simulink model "Engine"  (Simulink 9.3)
settings: Solver=ode23tb  StartTime=0.0  StopTime=50  FixedStep=0.001  EnableMultiTasking=on
values from neighbouring files (symbols this model uses):
  toggle_paf = toggle(2)    [RunEngine.m]
  toggle_vol = toggle(3)    [RunEngine.m]
  toggle_Waf = toggle(4)    [RunEngine.m]
  toggle_Wc = toggle(5)    [RunEngine.m]
  toggle_Wic = toggle(6)    [RunEngine.m]
  toggle_Wth = toggle(7)    [RunEngine.m]
  toggle_xth = toggle(8)    [RunEngine.m]
  toggle_ypic = toggle(9)    [RunEngine.m]
  toggle_ypim = toggle(10)    [RunEngine.m]
  toggle_yTic = toggle(11)    [RunEngine.m]
  toggle_yWaf = toggle(12)    [RunEngine.m]
undefined symbols (not defined in the file or in its folder): a0, a1, a2, dP_thrREF, KpThr, KpWg, n_r, Newton, r_c, Raphson, T_z, TC_ENGINE, TiThr, TiWg
libraries: simulink x3
(part 3 of 3)

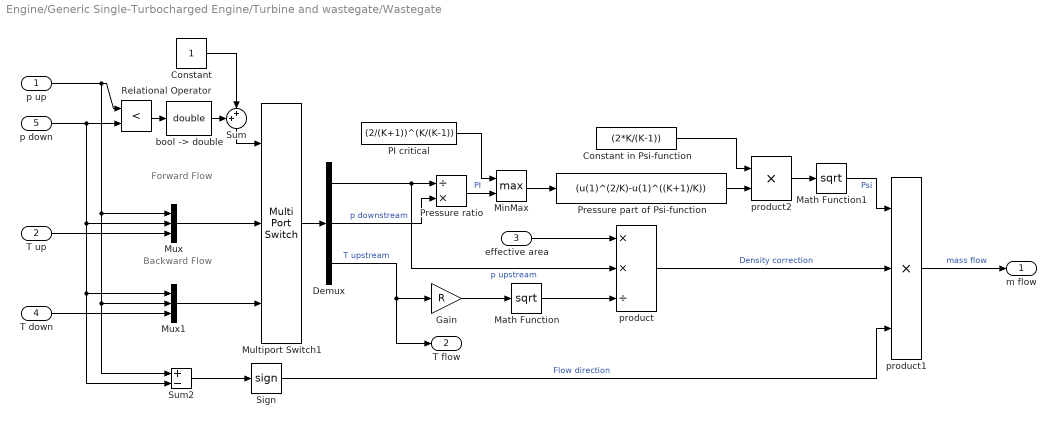
== system Engine/Generic Single-Turbocharged Engine/Turbine and wastegate/Wastegate ==
  note: Forward
      | Flow
  note: Backward
      | Flow
  p up : Inport
  T up : Inport  Port=2
  effective area : Inport  Port=3
  T down : Inport  Port=4
  p down : Inport  Port=5
  Constant : Constant
  Constant in Psi-function : Constant  Value=(2*K/(K-1))
  Demux : Demux  Outputs=3
  Gain : Gain  Gain=R  SaturateOnIntegerOverflow=on  OutDataTypeStr=Inherit: Same as input  ParamDataTypeStr=Inherit: Same as input
  Math Function : Math  Operator=sqrt  SaturateOnIntegerOverflow=on
  Math Function1 : Math  Operator=sqrt  SaturateOnIntegerOverflow=on
  MinMax : MinMax  Function=max  Inputs=2  ZeroCross=off  SaturateOnIntegerOverflow=on  InputSameDT=on
  Multiport Switch1 : MultiPortSwitch  Inputs=2  SaturateOnIntegerOverflow=on  InputSameDT=on
  Mux : Mux  Inputs=3
  Mux1 : Mux  Inputs=3
  PI critical : Constant  Value=(2/(K+1))^(K/(K-1))
  Pressure ratio : Product  Inputs=/*  SaturateOnIntegerOverflow=on  InputSameDT=on  OutDataTypeStr=Inherit: Same as first input
  Pressure part of Psi-function : Fcn  Expr=(u(1)^(2/K)-u(1)^((K+1)/K))
  Relational Operator : RelationalOperator  Operator=<  RndMeth=Nearest  InputSameDT=on
  Sign : Signum  ZeroCross=off
  Sum : Sum  Inputs=++|  SaturateOnIntegerOverflow=on  InputSameDT=on  OutDataTypeStr=Inherit: Same as first input
  Sum2 : Sum  Inputs=+-  SaturateOnIntegerOverflow=on  InputSameDT=on  OutDataTypeStr=Inherit: Same as first input
  "bool -> double" : DataTypeConversion  OutDataTypeStr=double  SaturateOnIntegerOverflow=on  RndMeth=Zero
  product : Product  Inputs=**/  SaturateOnIntegerOverflow=on  InputSameDT=on  OutDataTypeStr=Inherit: Same as first input
  product1 : Product  Inputs=3  SaturateOnIntegerOverflow=on  InputSameDT=on  OutDataTypeStr=Inherit: Same as first input
  product2 : Product  SaturateOnIntegerOverflow=on  InputSameDT=on  OutDataTypeStr=Inherit: Same as first input
  m flow : Outport
  T flow : Outport  Port=2
  wires:
  "bool -> double"/1 -> Sum/1
  Demux/3 -> T flow/1, Gain/1  "T upstream"
  Math Function1/1 -> product1/1  "Psi"
  product2/1 -> Math Function1/1
  Sign/1 -> product1/3  "Flow direction"
  product/1 -> product1/2  "Density correction"
  Pressure part of Psi-function/1 -> product2/2
  Constant in Psi-function/1 -> product2/1
  Math Function/1 -> product/3
  Gain/1 -> Math Function/1
  Demux/1 -> product/2, Pressure ratio/1  "p upstream"
  effective area/1 -> product/1
  product1/1 -> m flow/1  "mass flow"
  MinMax/1 -> Pressure part of Psi-function/1
  PI critical/1 -> MinMax/1
  Pressure ratio/1 -> MinMax/2  "PI"
  Sum2/1 -> Sign/1
  Demux/2 -> Pressure ratio/2  "p downstream"
  p up/1 -> Sum2/1, Mux1/2, Mux/1, Relational Operator/1
  p down/1 -> Sum2/2, Mux1/1, Mux/2, Relational Operator/2
  T up/1 -> Mux/3
  T down/1 -> Mux1/3
  Mux/1 -> Multiport Switch1/2
  Sum/1 -> Multiport Switch1/1
  Constant/1 -> Sum/2
  Mux1/1 -> Multiport Switch1/3
  Multiport Switch1/1 -> Demux/1
  Relational Operator/1 -> "bool -> double"/1

== system Engine/Generic Single-Turbocharged Engine/Compressor/Compressor Example/Compressor Efficiency ==
  w_c [rad/s] : Inport
  W_c [kg/s] : Inport  Port=2
  p_in [Pa] : Inport  Port=3
  T_in [K] : Inport  Port=4
  "Compressor Phi -> eta_c Parabola model" : Subsystem  mask(Compressor Efficiency){eta_max=TC_ENGINE.compressor.eta_max, Phi_max=TC_ENGINE.compressor.Phi_at_eta_max, eta_min=TC_ENGINE.compressor.minEfficiency}
      mask prompts: eta_max "Maximum efficiency [-]"; Phi_max "Phi at max efficiency [-]"; eta_min "Minimum efficiency [-]"
      mask help:
      | Calculates the compressor efficiency based on a simple
      | quadratic function in Phi. The maximum efficiency is
      | attained at a certain Phi, the curve is selected so that
      | Phi=0 gives eta=0. A minimum value of the efficiency can
      | also be given however it will always be bigger than
      | 1e-3, which is hardcoded into the model.
      |
      | The quadratic shape is a simple but yet powerful model
      | describing the data in Figure 10 in Eriksson (2007).
  "W_c -> Phi" : Subsystem  mask(Dimensionless Compressible Flow Parameter, Phi){D=TC_ENGINE.compressor.D, R=TC_ENGINE.gasProp.air.R}
      mask prompts: D "Compressor Diameter, D [m]"; R "Ideal gas constant, R [J/kg K]"
      mask help:
      | Calculation of the dimensionless compressible flow
      | parameter Phi, according to
      | Phi=Wc/(rho N D^3).
      mask Help:
      | Provide the parameter values for the:
      | compressor diameter D
      | and ideal gas constant R
      | and the block calculates the compressible dimensionless
      | flow parameter Phi.
  "rad/s -> rps" : Gain  Gain=1/2/pi
  eta_c : Outport
  wires:
  "rad/s -> rps"/1 -> "W_c -> Phi"/1(N_c [rps])
  w_c [rad/s]/1 -> "rad/s -> rps"/1
  "W_c -> Phi"/1(Phi) -> "Compressor Phi -> eta_c Parabola model"/1(Phi)
  W_c [kg/s]/1 -> "W_c -> Phi"/4(W_c)
  T_in [K]/1 -> "W_c -> Phi"/3(T_in)
  p_in [Pa]/1 -> "W_c -> Phi"/2(p_in)
  "Compressor Phi -> eta_c Parabola model"/1(eta_c) -> eta_c/1

== system Engine/Generic Single-Turbocharged Engine/Compressor/Compressor Example/Compressor Mass Flow ==
  w_c [rad/s] : Inport
  p_in [Pa] : Inport  Port=2
  T_in [K] : Inport  Port=3
  p_c [Pa] : Inport  Port=4
  Compressible Psi : Subsystem  mask(Calculation of Compressible Head Parameter){D=TC_ENGINE.compressor.D, gamma=TC_ENGINE.gasProp.air.kappa, c_p=TC_ENGINE.gasProp.air.cp}
      mask prompts: D "Compressor Diameter, D [m]"; gamma "Ratio of Specific Heats, gamma [-]"; c_p "Specific Heat, c_p [J/kg K]"
      mask help: Calculates the dimensionless head parameter Psi.
      mask Help:
      | Enter the parameter values:
      | -compressor diameter, D
      | -ratio of specific heats, gamma
      | -specific heat, c_p
      | and the block calculates the dimensionless compressible
      | head parameter from the input.
  "Compressor Psi -> Phi Elipse" : Subsystem  mask(Compressor Flow calculation){Psi_max=TC_ENGINE.compressor.Psi_max, Phi_max=TC_ENGINE.compressor.Phi_max}
      mask prompts: Psi_max "Maximum Psi [-]"; Phi_max "Maximum Phi [-]"
      mask help:
      | Calculates the dimensionless flow variable from the
      | dimensionless head parameter according to the elipse
      | model from Eriksson (2007).
      mask Help:
      | Enter the maximum flow and head parameter values that
      | determine the edges of the elipse.
  "Phi -> W_c" : Subsystem  mask(Mass Flow from Phi){D=TC_ENGINE.compressor.D, R=TC_ENGINE.gasProp.air.R}
      mask prompts: D "Compressor Diameter, D [m]"; R "Ideal Gas Constant, R [J/kg K]"
      mask help:
      | Calculates compressor mass flow from the compressible
      | dimensionless flow parameter Phi.
      mask Help:
      | Provide the following parameters,
      | compressor diameter, D
      | and ideal gas constant, R
      | and the block calculates the compressor mass flow from
      | the inputs.
  "rad/s -> rps" : Gain  Gain=1/2/pi
  W_c : Outport
  wires:
  p_in [Pa]/1 -> "Phi -> W_c"/2(p_in), Compressible Psi/2(p_in [Pa])
  T_in [K]/1 -> "Phi -> W_c"/3(T_in), Compressible Psi/3(T_in [K])
  p_c [Pa]/1 -> Compressible Psi/4(p_c [Pa])
  Compressible Psi/1(Psi) -> "Compressor Psi -> Phi Elipse"/1(Psi)
  "Phi -> W_c"/1(W_c) -> W_c/1
  w_c [rad/s]/1 -> "rad/s -> rps"/1
  "rad/s -> rps"/1 -> "Phi -> W_c"/1(N_c [rps]), Compressible Psi/1(N_c [rps])
  "Compressor Psi -> Phi Elipse"/1(Phi) -> "Phi -> W_c"/4(Phi)

== system Engine/Generic Single-Turbocharged Engine/Compressor/Compressor Example/Compressor Temperature ==
  eta_c : Inport
  T_in : Inport  Port=2
  Pi_c : Inport  Port=3
  Add : Sum
  Add1 : Sum  Inputs=+-
  Constant : Constant  Value=1-1/gamma_c
  Constant1 : Constant
  Constant2 : Constant
  Divide1 : Product  Inputs=*/
  Math Function : Math  Operator=pow  SaturateOnIntegerOverflow=on
  Mult : Product
  T_out : Outport
  wires:
  Constant/1 -> Math Function/2
  Constant1/1 -> Add1/2
  eta_c/1 -> Divide1/2
  Add1/1 -> Divide1/1
  Math Function/1 -> Add1/1
  Constant2/1 -> Add/2
  Mult/1 -> T_out/1
  Pi_c/1 -> Math Function/1
  T_in/1 -> Mult/1
  Add/1 -> Mult/2
  Divide1/1 -> Add/1

== system Engine/Generic Single-Turbocharged Engine/Compressor/Compressor Example/Compressor Torque ==
  omega_c : Inport
  mFlow_c : Inport  Port=2
  T_in : Inport  Port=3
  T_out : Inport  Port=4
  Add1 : Sum  Inputs=+-
  Constant : Constant  Value=0
  Divide2 : Product  Inputs=**/
  MinMax : MinMax  Function=max  Inputs=2  ZeroCross=off
  cp_inlet : Gain  Gain=c_p
  Tq_c : Outport
  wires:
  cp_inlet/1 -> Tq_c/1  "Tq_c"
  Divide2/1 -> cp_inlet/1
  Add1/1 -> MinMax/2
  MinMax/1 -> Divide2/1
  Constant/1 -> MinMax/1
  T_out/1 -> Add1/1
  T_in/1 -> Add1/2
  mFlow_c/1 -> Divide2/2
  omega_c/1 -> Divide2/3

== system Engine/Generic Single-Turbocharged Engine/Compressor/Compressor Example/PI-calc ==
  p_af : Inport
  p_c : Inport  Port=2
  Constant2 : Constant
  MinMax : MinMax  Function=max  Inputs=2  ZeroCross=off  SaturateOnIntegerOverflow=on  InputSameDT=on
  Product2 : Product  Inputs=/*  SaturateOnIntegerOverflow=on  OutDataTypeStr=Inherit: Same as first input
  PI : Outport
  wires:
  MinMax/1 -> PI/1
  p_c/1 -> Product2/2
  p_af/1 -> Product2/1
  Constant2/1 -> MinMax/2
  Product2/1 -> MinMax/1

== system Engine/Generic Single-Turbocharged Engine/Engine/Engine flow/Volumetric Efficiency Fault ==
  Cvol : Inport
  Pulse Generator : DiscretePulseGenerator  PulseType=Time based  Period=150  PulseWidth=20  PhaseDelay=30
  Sum : Sum  Inputs=|+-
  To Workspace26 : ToWorkspace  VariableName=fCvolSig  SaveFormat=Timeseries  SampleTime=-1
  "toggle " : Gain  Gain=toggle_vol*0.08  SaturateOnIntegerOverflow=on  OutDataTypeStr=Inherit: Same as input  ParamDataTypeStr=Inherit: Same as input
  fCvol : Outport
  wires:
  Cvol/1 -> Sum/1
  "toggle "/1 -> To Workspace26/1, Sum/2
  Pulse Generator/1 -> "toggle "/1
  Sum/1 -> fCvol/1

== system Engine/Generic Single-Turbocharged Engine/Engine/Exhaust temperature drop Model 1/Selector for correlation constants ==
  Blair : Constant  Value=[0.02 0.8 0 0]
  Caton Heywwod : Constant  Value=[0.258 0.8 0 0]
  DOHC Downpipe : Constant  Value=[0.26 0.6 0 0]
  Eriksson : Constant  Value=[0.48 0.5 0 0]
  Malcow et al : Constant  Value=[0.0483 0.783 0 0]
  Meisner Sorenson : Constant  Value=[0.26 0.6 0 0]
  Multiport Switch : MultiPortSwitch  Inputs=17  SaturateOnIntegerOverflow=on  InputSameDT=on
  PROMEX : Constant  Value=[0.027 0.82 0 0]
  Reynolds : Constant  Value=[0.0175 1 0 0]
  Selector : Constant  Value=corrSelector
  Shayler 1997a : Constant  Value=[0.18 0.7 0 0]
  Sieder Tate : Constant  Value=[0.027 0.8 0.3333 0.14]
  Standard : Constant  Value=[0.01994 0.8 0 0]
  Valencia downpipe : Constant  Value=[0.83 0.46 0 0]
  Wendland Takedown : Constant  Value=[0.081 0.8 0.3333 0.14]
  Wendland tailpipe : Constant  Value=[0.0432 0.8 0.3333 0.14]
  Woods : Constant  Value=[0.02948 0.8 0 0]
  standard laminar 2 : Constant  Value=[1.86 0.333 0.333 0.14]
  standard turbulent : Constant  Value=[0.023 0.8 0.3 0]
  Correlation Constants : Outport
  wires:
  Meisner Sorenson/1 -> Multiport Switch/2
  Caton Heywwod/1 -> Multiport Switch/8
  Reynolds/1 -> Multiport Switch/18
  standard laminar 2/1 -> Multiport Switch/17
  Eriksson/1 -> Multiport Switch/16
  standard turbulent/1 -> Multiport Switch/15
  Standard/1 -> Multiport Switch/14
  Blair/1 -> Multiport Switch/13
  Woods/1 -> Multiport Switch/12
  PROMEX/1 -> Multiport Switch/11
  Valencia downpipe/1 -> Multiport Switch/10
  DOHC Downpipe/1 -> Multiport Switch/9
  Malcow et al/1 -> Multiport Switch/7
  Wendland tailpipe/1 -> Multiport Switch/6
  Wendland Takedown/1 -> Multiport Switch/5
  Shayler 1997a/1 -> Multiport Switch/3
  Multiport Switch/1 -> Correlation Constants/1
  Selector/1 -> Multiport Switch/1
  Sieder Tate/1 -> Multiport Switch/4

== system Engine/Generic Single-Turbocharged Engine/Turbine and wastegate/Turbine1/Turbine Temperature ==
  eta_t : Inport
  T_in : Inport  Port=2
  Pi_t : Inport  Port=3
  (gamma-1)/gamma : Constant  Value=1-1/gamma
  Add : Sum  Inputs=+-
  Add1 : Sum  Inputs=+-
  Constant : Constant
  Divide2 : Product  Inputs=**
  Divide3 : Product  Inputs=**
  Math Function : Math  Operator=pow  SaturateOnIntegerOverflow=on
  T_out : Outport
  wires:
  eta_t/1 -> Divide2/2
  T_in/1 -> Divide3/2
  Divide3/1 -> T_out/1
  Constant/1 -> Add/1, Add1/1
  Math Function/1 -> Add/2
  Add/1 -> Divide2/1
  Pi_t/1 -> Math Function/1
  (gamma-1)/gamma/1 -> Math Function/2
  Divide2/1 -> Add1/2
  Add1/1 -> Divide3/1

== system Engine/Generic Single-Turbocharged Engine/Turbine and wastegate/Turbine1/Turbine Torque ==
  omega_t : Inport
  mFlow_t : Inport  Port=2
  T_in : Inport  Port=3
  T_out : Inport  Port=4
  Add : Sum  Inputs=+-
  Constant : Constant  Value=0
  Divide2 : Product  Inputs=**/
  MinMax : MinMax  Function=max  Inputs=2  ZeroCross=off
  cp_eg : Gain  Gain=c_p
  Tq_t : Outport
  wires:
  Divide2/1 -> cp_eg/1
  cp_eg/1 -> Tq_t/1  "Tq_t"
  Add/1 -> MinMax/2
  MinMax/1 -> Divide2/1
  Constant/1 -> MinMax/1
  T_in/1 -> Add/1
  T_out/1 -> Add/2
  mFlow_t/1 -> Divide2/2
  omega_t/1 -> Divide2/3

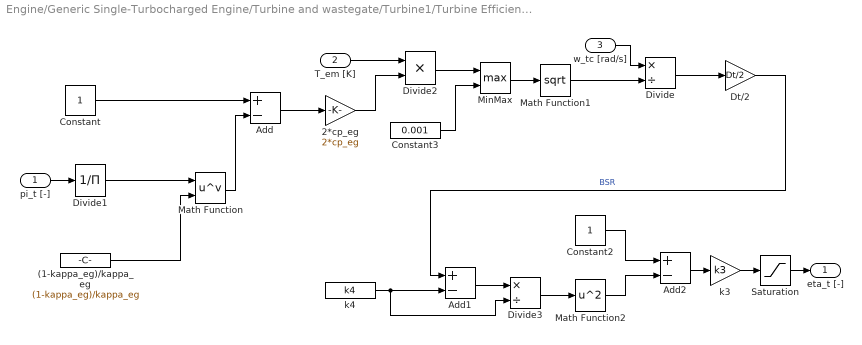
== system Engine/Generic Single-Turbocharged Engine/Turbine and wastegate/Turbine1/Turbine Efficiency ==
  pi_t [-] : Inport
  T_em [K] : Inport  Port=2
  w_tc [rad/s] : Inport  Port=3
  (1-kappa_eg)/kappa_eg : Constant  Value=(1-kappa_eg)/kappa_eg
  2*cp_eg : Gain  Gain=2*cp_eg
  Add : Sum  Inputs=+-
  Add1 : Sum  Inputs=+-
  Add2 : Sum  Inputs=+-
  Constant : Constant
  Constant2 : Constant
  Constant3 : Constant  Value=0.001
  Divide : Product  Inputs=*/
  Divide1 : Product  Inputs=/
  Divide2 : Product  Inputs=**
  Divide3 : Product  Inputs=*/
  Dt/2 : Gain  Gain=Dt/2
  Math Function : Math  Operator=pow  SaturateOnIntegerOverflow=on
  Math Function1 : Math  Operator=sqrt  SaturateOnIntegerOverflow=on
  Math Function2 : Math  Operator=square  SaturateOnIntegerOverflow=on
  MinMax : MinMax  Function=max  Inputs=2  ZeroCross=off
  Saturation : Saturate  UpperLimit=k3  LowerLimit=turbMinEff  ZeroCross=off
  k3 : Gain  Gain=k3
  k4 : Constant  Value=k4
  eta_t [-] : Outport
  wires:
  Saturation/1 -> eta_t [-]/1
  (1-kappa_eg)/kappa_eg/1 -> Math Function/2
  Dt/2/1 -> Add1/1  "BSR"
  Constant/1 -> Add/1
  Math Function/1 -> Add/2
  Add/1 -> 2*cp_eg/1
  Math Function1/1 -> Divide/2
  2*cp_eg/1 -> Divide2/2
  Divide2/1 -> MinMax/1
  Constant3/1 -> MinMax/2
  MinMax/1 -> Math Function1/1
  Divide/1 -> Dt/2/1
  k4/1 -> Add1/2, Divide3/2
  Add1/1 -> Divide3/1
  Divide3/1 -> Math Function2/1
  Constant2/1 -> Add2/1
  Math Function2/1 -> Add2/2
  Add2/1 -> k3/1
  T_em [K]/1 -> Divide2/1
  w_tc [rad/s]/1 -> Divide/1
  pi_t [-]/1 -> Divide1/1
  k3/1 -> Saturation/1
  Divide1/1 -> Math Function/1

== system Engine/Generic Single-Turbocharged Engine/Turbine and wastegate/Turbine1/Turbine Pressure ratio ==
  p_t [Pa] : Inport
  p_em [Pa] : Inport  Port=2
  Constant : Constant
  Divide : Product  Inputs=*/
  MinMax : MinMax  Inputs=2  ZeroCross=off
  pi_t [-] : Outport
  wires:
  Divide/1 -> MinMax/2
  Constant/1 -> MinMax/1
  p_t [Pa]/1 -> Divide/1
  MinMax/1 -> pi_t [-]/1
  p_em [Pa]/1 -> Divide/2

== system Engine/Generic Single-Turbocharged Engine/Turbine and wastegate/Turbine1/Turbine mass flow ==
  pi_t : Inport
  p_em [Pa] : Inport  Port=2
  T_em : Inport  Port=3
  Constant : Constant  Value=k2
  Constant2 : Constant
  Constant4 : Constant  Value=0
  Divide : Product  Inputs=*/*
  Gain : Gain  Gain=k1
  Math Function : Math  Operator=sqrt  SaturateOnIntegerOverflow=on
  Math Function1 : Math  Operator=pow  SaturateOnIntegerOverflow=on
  Math Function2 : Math  Operator=sqrt  SaturateOnIntegerOverflow=on
  MinMax : MinMax  Function=max  Inputs=2  ZeroCross=off
  Sum : Sum  Inputs=|+-
  W_t : Outport
  wires:
  Constant2/1 -> Sum/1
  Math Function1/1 -> Sum/2
  Constant/1 -> Math Function1/2
  Constant4/1 -> MinMax/2
  Sum/1 -> MinMax/1
  Math Function/1 -> Gain/1
  Gain/1 -> Divide/1
  Math Function2/1 -> Divide/2
  Divide/1 -> W_t/1
  p_em [Pa]/1 -> Divide/3
  pi_t/1 -> Math Function1/1
  MinMax/1 -> Math Function/1
  T_em/1 -> Math Function2/1

== system Engine/Generic Single-Turbocharged Engine/Compressor/Compressor Example/Compressor Efficiency/Compressor Phi -> eta_c Parabola model ==
  Phi : Inport
  Constant1 : Constant  Value=eta_max
  Constant2 : Constant  Value=Phi_max
  Gain1 : Gain  Gain=2
  Product : Product  Inputs=3  RndMeth=Zero
  Product1 : Product  Inputs=//*  RndMeth=Zero
  Saturation : Saturate  UpperLimit=1  LowerLimit=max(eta_min,1e-3)  ZeroCross=off
  Sum : Sum  Inputs=|-+
  eta_c : Outport
  wires:
  Constant2/1 -> Gain1/1, Product1/1, Product1/2
  Phi/1 -> Product/1, Sum/1
  Gain1/1 -> Sum/2
  Sum/1 -> Product/2
  Constant1/1 -> Product1/3
  Product1/1 -> Product/3
  Product/1 -> Saturation/1
  Saturation/1 -> eta_c/1

== system Engine/Generic Single-Turbocharged Engine/Compressor/Compressor Example/Compressor Efficiency/W_c -> Phi ==
  N_c [rps] : Inport
  p_in : Inport  Port=2
  T_in : Inport  Port=3
  W_c : Inport  Port=4
  Constant1 : Constant  Value=D^3
  Constant2 : Constant  Value=R
  Divide2 : Product  Inputs=*//
  Mult : Product  Inputs=*///
  Phi : Outport
  wires:
  Constant1/1 -> Mult/4
  N_c [rps]/1 -> Mult/3
  Divide2/1 -> Mult/2
  W_c/1 -> Mult/1
  Constant2/1 -> Divide2/3
  T_in/1 -> Divide2/2
  p_in/1 -> Divide2/1
  Mult/1 -> Phi/1

== system Engine/Generic Single-Turbocharged Engine/Compressor/Compressor Example/Compressor Mass Flow/Compressible Psi ==
  N_c [rps] : Inport
  p_in [Pa] : Inport  Port=2
  T_in [K] : Inport  Port=3
  p_c [Pa] : Inport  Port=4
  Add : Sum  Inputs=+-
  Constant : Constant
  Constant1 : Constant  Value=(gamma-1)/gamma
  Constant2 : Constant  Value=c_p
  Constant3 : Constant  Value=D^2
  Divide : Product  Inputs=*/
  Divide1 : Product  Inputs=*/
  Divide2 : Product  Inputs=***/
  Math Function : Math  Operator=pow  SaturateOnIntegerOverflow=on
  Math Function1 : Math  Operator=square  SaturateOnIntegerOverflow=on
  Saturation : Saturate  UpperLimit=10  LowerLimit=1  ZeroCross=off
  Psi : Outport
  wires:
  p_c [Pa]/1 -> Divide/1
  p_in [Pa]/1 -> Divide/2
  Divide/1 -> Saturation/1
  Constant1/1 -> Math Function/2
  Math Function/1 -> Add/1
  Constant/1 -> Add/2
  T_in [K]/1 -> Divide2/2
  Add/1 -> Divide2/3
  Divide2/1 -> Psi/1
  Saturation/1 -> Math Function/1
  Constant2/1 -> Divide1/1
  Constant3/1 -> Divide1/2
  Divide1/1 -> Divide2/1
  N_c [rps]/1 -> Math Function1/1
  Math Function1/1 -> Divide2/4

== system Engine/Generic Single-Turbocharged Engine/Compressor/Compressor Example/Compressor Mass Flow/Compressor Psi -> Phi Elipse ==
  Psi : Inport
  Add : Sum  Inputs=-+
  Constant : Constant
  Gain : Gain  Gain=1/Psi_max
  Gain1 : Gain  Gain=Phi_max
  Math Function : Math  Operator=square  SaturateOnIntegerOverflow=on
  Math Function1 : Math  Operator=sqrt  SaturateOnIntegerOverflow=on
  Saturation : Saturate  UpperLimit=1  LowerLimit=0  ZeroCross=off
  Phi : Outport
  wires:
  Math Function1/1 -> Gain1/1
  Gain1/1 -> Phi/1
  Psi/1 -> Gain/1
  Gain/1 -> Math Function/1
  Saturation/1 -> Add/1
  Math Function/1 -> Saturation/1
  Add/1 -> Math Function1/1
  Constant/1 -> Add/2

== system Engine/Generic Single-Turbocharged Engine/Compressor/Compressor Example/Compressor Mass Flow/Phi -> W_c ==
  N_c [rps] : Inport
  p_in : Inport  Port=2
  T_in : Inport  Port=3
  Phi : Inport  Port=4
  Constant1 : Constant  Value=D^3
  Constant2 : Constant  Value=R
  Divide2 : Product  Inputs=*//
  Mult : Product  Inputs=4
  W_c : Outport
  wires:
  Mult/1 -> W_c/1
  p_in/1 -> Divide2/1
  T_in/1 -> Divide2/2
  Constant2/1 -> Divide2/3
  Phi/1 -> Mult/1
  Divide2/1 -> Mult/2
  N_c [rps]/1 -> Mult/3
  Constant1/1 -> Mult/4
